simulink model "test_for_flighttests"  (R2018a)
settings: Solver=VariableStepAuto  StartTime=0.0  StopTime=50  MaxStep=1  MinStep=.005  RelTol=10  AbsTol=10
undefined symbols (not defined in the file or in its folder): Angular, Linear, state
libraries: robotlib x11, vrlib x1
settings Model: EnablePacing=on  Creator=lenny  LastModifiedBy=lenny
settings SolverCC: MaxConsecutiveMinStep=999999  ShapePreserveControl=EnableAll

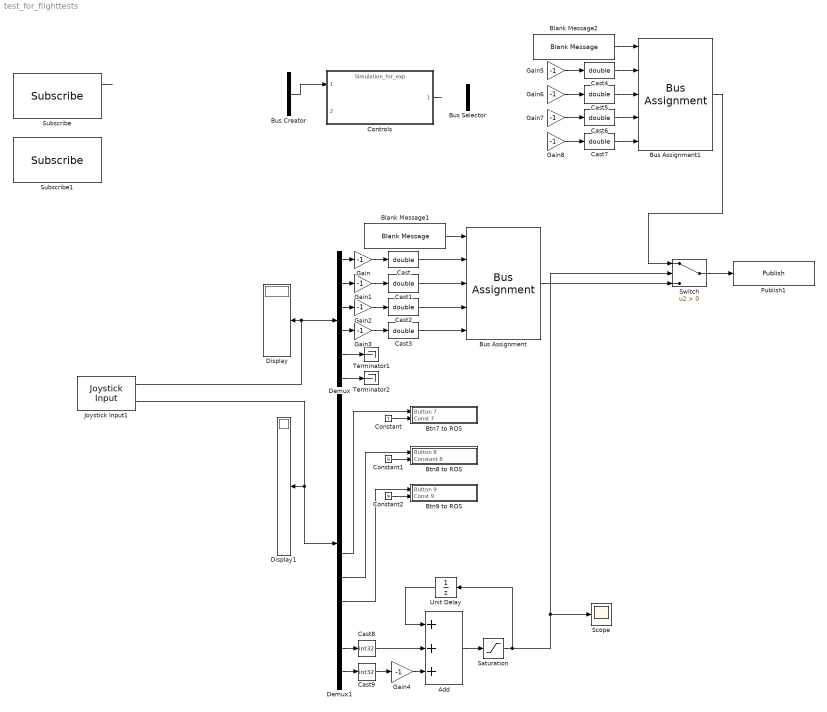
== system test_for_flighttests ==
  Add : Sum  Inputs=+++
  Blank Message1 : robotlib/Blank Message  SourceLibraryInfo=This block requires Robotics System Toolbox  messageType=geometry_msgs/Twist  SampleTime=inf
      settings: SourceProductBaseCode=RO
  Blank Message2 : robotlib/Blank Message  SourceLibraryInfo=This block requires Robotics System Toolbox  messageType=geometry_msgs/Twist  SampleTime=inf
      settings: SourceProductBaseCode=RO
  Btn7 to ROS : Subsystem
  Btn8 to ROS : Subsystem
  Btn9 to ROS : Subsystem
  Bus Assignment : BusAssignment  AssignedSignals=Linear.Y,Linear.X,Angular.Z,Linear.Z
  Bus Assignment1 : BusAssignment  AssignedSignals=Linear.Y,Linear.X,Angular.Z,Linear.Z
  Bus Creator : BusCreator  Inputs=state.vel,state.eul,state.pos
  Bus Selector : BusSelector  OutputSignals=signal1,signal2
  Cast{,1..7} (8 alike) : DataTypeConversion  OutDataTypeStr=double
  Cast8 : DataTypeConversion  OutDataTypeStr=int32
  Cast9 : DataTypeConversion  OutDataTypeStr=int32
  Constant : Constant  Value=7
  Constant1 : Constant  Value=8
  Constant2 : Constant  Value=9
  Controls : ModelReference  ModelNameDialog=Simulation_for_exp.slx  SimulationMode=Normal  ModelReferenceVersion=1.277
  Demux : Demux  Outputs=6
  Demux1 : Demux  Outputs=12
  Display : Display
  Display1 : Display
  Gain{,1..8} (9 alike) : Gain  Gain=-1
  Joystick Input1 : vrlib/Joystick Input  joyid=1  adjustports=on  forcefeed=off
      settings: SourceProductBaseCode=VR
  Publish1 : robotlib/Publish  SourceLibraryInfo=This block requires Robotics System Toolbox  topicSource=Specify your own  topic=/bebop/cmd_vel  messageType=geometry_msgs/Twist  messageQueueLength=1
      settings: SourceProductBaseCode=RO
  Saturation : Saturate  UpperLimit=1  LowerLimit=0
  Scope : Scope
  Subscribe : robotlib/Subscribe  SourceLibraryInfo=This block requires Robotics System Toolbox  topicSource=Specify your own  topic=/bebop/odom  messageType=nav_msgs/Odometry  sampleTime=-1  messageQueueLength=1
      settings: SourceProductBaseCode=RO
  Subscribe1 : robotlib/Subscribe  SourceLibraryInfo=This block requires Robotics System Toolbox  topicSource=Select from ROS network  topic=/my_topic  messageType=geometry_msgs/Point  sampleTime=-1  messageQueueLength=1
      settings: SourceProductBaseCode=RO
  Switch : Switch  Criteria=u2 > Threshold
  Terminator1 : Terminator
  Terminator2 : Terminator
  Unit Delay : UnitDelay  SampleTime=-1
  wires:
  Demux/6 -> Terminator2/1
  Demux/5 -> Terminator1/1
  Joystick Input1/2 -> Demux1/1, Display1/1
  Joystick Input1/1 -> Display/1, Demux/1
  Constant/1 -> Btn7 to ROS/2(Const 7)
  Demux1/7 -> Btn7 to ROS/1(Button 7)
  Constant1/1 -> Btn8 to ROS/2(Constant 8)
  Demux1/8 -> Btn8 to ROS/1(Button 8)
  Constant2/1 -> Btn9 to ROS/2(Const 9)
  Demux1/9 -> Btn9 to ROS/1(Button 9)
  Bus Assignment/1 -> Switch/3
  Blank Message1/1 -> Bus Assignment/1
  Demux/1 -> Gain/1
  Demux/2 -> Gain1/1
  Demux/4 -> Gain3/1
  Demux/3 -> Gain2/1
  Gain/1 -> Cast/1
  Gain1/1 -> Cast1/1
  Gain2/1 -> Cast2/1
  Gain3/1 -> Cast3/1
  Switch/1 -> Publish1/1
  Cast1/1 -> Bus Assignment/3
  Cast/1 -> Bus Assignment/2
  Cast2/1 -> Bus Assignment/4
  Cast3/1 -> Bus Assignment/5
  Demux1/12 -> Cast9/1
  Demux1/11 -> Cast8/1
  Gain4/1 -> Add/3
  Add/1 -> Saturation/1
  Saturation/1 -> Unit Delay/1, Scope/1, Switch/2
  Unit Delay/1 -> Add/1
  Bus Assignment1/1 -> Switch/1
  Cast6/1 -> Bus Assignment1/4
  Blank Message2/1 -> Bus Assignment1/1
  Cast4/1 -> Bus Assignment1/2
  Gain7/1 -> Cast6/1
  Cast7/1 -> Bus Assignment1/5
  Gain8/1 -> Cast7/1
  Gain5/1 -> Cast4/1
  Gain6/1 -> Cast5/1
  Cast5/1 -> Bus Assignment1/3
  Cast8/1 -> Add/2
  Cast9/1 -> Gain4/1
  ? -> Gain5/1
  ? -> Gain6/1
  ? -> Gain7/1
  ? -> Gain8/1
  Controls/1 -> ?
  Bus Creator/1 -> Controls/1
  Subscribe/1 -> ?

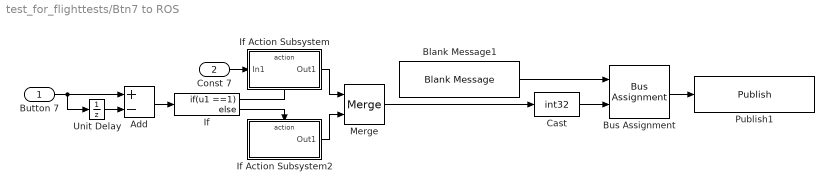
== system test_for_flighttests/Btn7 to ROS ==
  Button 7 : Inport
  Const 7 : Inport  Port=2
  Add : Sum  Inputs=+-
  Blank Message1 : robotlib/Blank Message  SourceLibraryInfo=This block requires Robotics System Toolbox  messageType=std_msgs/Int32  SampleTime=inf
      settings: SourceProductBaseCode=RO
  Bus Assignment : BusAssignment  AssignedSignals=Data
  Cast : DataTypeConversion  OutDataTypeStr=int32
  If : If  IfExpression=u1 ==1
  If Action Subsystem : Subsystem  TreatAsAtomicUnit=on
  If Action Subsystem2 : Subsystem  TreatAsAtomicUnit=on
  Merge : Merge
  Publish1 : robotlib/Publish  SourceLibraryInfo=This block requires Robotics System Toolbox  topicSource=Specify your own  topic=/auto/flt_st_cmd  messageType=std_msgs/Int32  messageQueueLength=1
      settings: SourceProductBaseCode=RO
  Unit Delay : UnitDelay  SampleTime=-1
  wires:
  If Action Subsystem/1(Out1) -> Merge/1
  If/1 -> If Action Subsystem/Action
  Blank Message1/1 -> Bus Assignment/1
  Button 7/1 -> Unit Delay/1, Add/1
  If/2 -> If Action Subsystem2/Action
  Bus Assignment/1 -> Publish1/1
  Add/1 -> If/1
  Merge/1 -> Cast/1
  Unit Delay/1 -> Add/2
  Const 7/1 -> If Action Subsystem/1(In1)
  If Action Subsystem2/1(Out1) -> Merge/2
  Cast/1 -> Bus Assignment/2

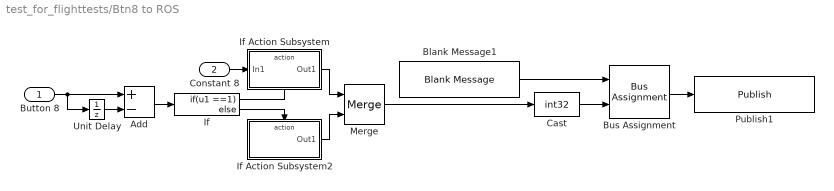
== system test_for_flighttests/Btn8 to ROS ==
  Button 8 : Inport
  Constant 8 : Inport  Port=2
  Add : Sum  Inputs=+-
  Blank Message1 : robotlib/Blank Message  SourceLibraryInfo=This block requires Robotics System Toolbox  messageType=std_msgs/Int32  SampleTime=inf
      settings: SourceProductBaseCode=RO
  Bus Assignment : BusAssignment  AssignedSignals=Data
  Cast : DataTypeConversion  OutDataTypeStr=int32
  If : If  IfExpression=u1 ==1
  If Action Subsystem : Subsystem  TreatAsAtomicUnit=on
  If Action Subsystem2 : Subsystem  TreatAsAtomicUnit=on
  Merge : Merge
  Publish1 : robotlib/Publish  SourceLibraryInfo=This block requires Robotics System Toolbox  topicSource=Specify your own  topic=/auto/flt_st_cmd  messageType=std_msgs/Int32  messageQueueLength=1
      settings: SourceProductBaseCode=RO
  Unit Delay : UnitDelay  SampleTime=-1
  wires:
  Bus Assignment/1 -> Publish1/1
  If/2 -> If Action Subsystem2/Action
  If Action Subsystem2/1(Out1) -> Merge/2
  Add/1 -> If/1
  If Action Subsystem/1(Out1) -> Merge/1
  Cast/1 -> Bus Assignment/2
  Constant 8/1 -> If Action Subsystem/1(In1)
  Blank Message1/1 -> Bus Assignment/1
  Button 8/1 -> Unit Delay/1, Add/1
  Merge/1 -> Cast/1
  If/1 -> If Action Subsystem/Action
  Unit Delay/1 -> Add/2

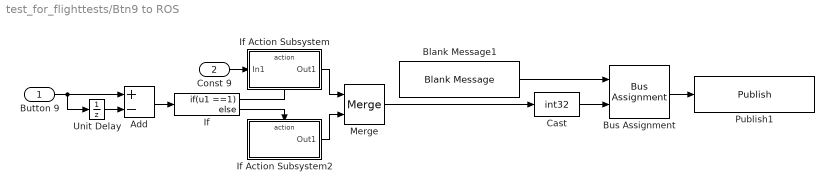
== system test_for_flighttests/Btn9 to ROS ==
  Button 9 : Inport
  Const 9 : Inport  Port=2
  Add : Sum  Inputs=+-
  Blank Message1 : robotlib/Blank Message  SourceLibraryInfo=This block requires Robotics System Toolbox  messageType=std_msgs/Int32  SampleTime=inf
      settings: SourceProductBaseCode=RO
  Bus Assignment : BusAssignment  AssignedSignals=Data
  Cast : DataTypeConversion  OutDataTypeStr=int32
  If : If  IfExpression=u1 ==1
  If Action Subsystem : Subsystem  TreatAsAtomicUnit=on
  If Action Subsystem2 : Subsystem  TreatAsAtomicUnit=on
  Merge : Merge
  Publish1 : robotlib/Publish  SourceLibraryInfo=This block requires Robotics System Toolbox  topicSource=Specify your own  topic=/auto/flt_st_cmd  messageType=std_msgs/Int32  messageQueueLength=1
      settings: SourceProductBaseCode=RO
  Unit Delay : UnitDelay  SampleTime=-1
  wires:
  Bus Assignment/1 -> Publish1/1
  If/2 -> If Action Subsystem2/Action
  If Action Subsystem2/1(Out1) -> Merge/2
  Add/1 -> If/1
  If Action Subsystem/1(Out1) -> Merge/1
  Cast/1 -> Bus Assignment/2
  Const 9/1 -> If Action Subsystem/1(In1)
  Blank Message1/1 -> Bus Assignment/1
  Button 9/1 -> Unit Delay/1, Add/1
  Merge/1 -> Cast/1
  If/1 -> If Action Subsystem/Action
  Unit Delay/1 -> Add/2

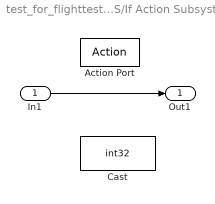
== system test_for_flighttests/Btn7 to ROS/If Action Subsystem ==
  In1 : Inport
  Action Port : ActionPort  ActionType=then
  Cast : DataTypeConversion  OutDataTypeStr=int32
  Out1 : Outport
  wires:
  In1/1 -> Out1/1

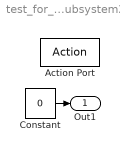
== system test_for_flighttests/Btn7 to ROS/If Action Subsystem2 ==
  Action Port : ActionPort  ActionType=else
  Constant : Constant  Value=0
  Out1 : Outport
  wires:
  Constant/1 -> Out1/1

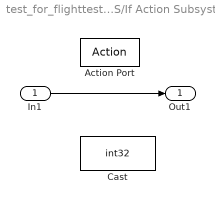
== system test_for_flighttests/Btn8 to ROS/If Action Subsystem ==
  In1 : Inport
  Action Port : ActionPort  ActionType=then
  Cast : DataTypeConversion  OutDataTypeStr=int32
  Out1 : Outport
  wires:
  In1/1 -> Out1/1

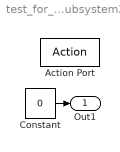
== system test_for_flighttests/Btn8 to ROS/If Action Subsystem2 ==
  Action Port : ActionPort  ActionType=else
  Constant : Constant  Value=0
  Out1 : Outport
  wires:
  Constant/1 -> Out1/1

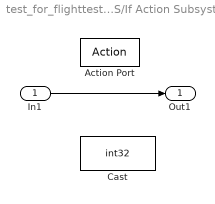
== system test_for_flighttests/Btn9 to ROS/If Action Subsystem ==
  In1 : Inport
  Action Port : ActionPort  ActionType=then
  Cast : DataTypeConversion  OutDataTypeStr=int32
  Out1 : Outport
  wires:
  In1/1 -> Out1/1

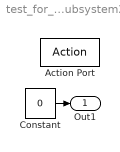
== system test_for_flighttests/Btn9 to ROS/If Action Subsystem2 ==
  Action Port : ActionPort  ActionType=else
  Constant : Constant  Value=0
  Out1 : Outport
  wires:
  Constant/1 -> Out1/1
